simulink model "ClosedLoop_sim"  (R2018b)
settings: Solver=VariableStepAuto  StartTime=0.0  StopTime=10.0  RelTol=1e-3
libraries: simulink x2
settings Model: Creator=manzand  LastModifiedBy=manzand

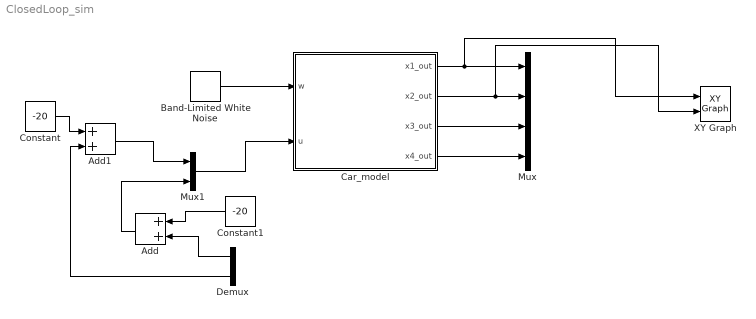
== system ClosedLoop_sim ==
  Add : Sum
  Add1 : Sum
  Band-Limited White Noise : simulink/Sources/Band-Limited White Noise  Cov=[10^-4]  Ts=0.01  seed=[23341]
  Car_model : Stateflow chart  TreatAsAtomicUnit=on
  Constant : Constant  Value=-20
  Constant1 : Constant  Value=-20
  Demux : Demux  Outputs=2
  Mux : Mux
  Mux1 : Mux  Inputs=2
  XY Graph : simulink/Sinks/XY Graph  xmin=-1  xmax=1  ymin=-1  ymax=1  st=-1
  wires:
  Band-Limited White Noise/1 -> Car_model/1(w)
  Car_model/1(x1_out) -> XY Graph/1, Mux/1
  Car_model/2(x2_out) -> XY Graph/2, Mux/2
  Car_model/3(x3_out) -> Mux/3
  Car_model/4(x4_out) -> Mux/4
  Mux1/1 -> Car_model/2(u)
  Constant1/1 -> Add/1
  Constant/1 -> Add1/1
  Add/1 -> Mux1/2
  Add1/1 -> Mux1/1
  Demux/1 -> Add/2
  Demux/2 -> Add1/2

== stateflow chart ClosedLoop_sim/Car_model ==
  settings: updateMethod=CONTINUOUS
  state Car_model
    du:
    x1_dot = x2;
    x2_dot = -x1 + 0.1*sin(x3);
    x3_dot = x(4);
    x4_dor = u;
    %OUTPUTS
    x1_out = x1;
    x2_out = x2;
    x3_out = x3;
    x4_out = x4;
  (default) -> Car_model : {x1 = 9.52;
      | x2 = -4.47;
      | x3 = 2.1;
      | x4 = 1.5;}
  data: x1_out output; x2_out output; x3_out output; x4_out output; x1 local; x2 local; x3 local; x4 local; w input; u input
  data x1 settings: updateMethod=SF_CONTINUOUS_TIME_DATA
  data x2 settings: updateMethod=SF_CONTINUOUS_TIME_DATA
  data x3 settings: updateMethod=SF_CONTINUOUS_TIME_DATA
  data x4 settings: updateMethod=SF_CONTINUOUS_TIME_DATA
